simulink model "process_model_simulink"  (R2014b)
settings: Solver=ode45  StartTime=0.0  StopTime=500  RelTol=1e-3
values from neighbouring files (symbols this model uses):
  gs11_d = double(coeff_gs11(1))    [fase_minima.m]    (also in fase_nao_minima.m; model_minimum_phase.m; model_nonminimum_phase.m)
  gs11_ds = double(coeff_gs11(2))    [fase_minima.m]    (also in fase_nao_minima.m; model_minimum_phase.m; model_nonminimum_phase.m)
  gs11_n = gamma1*c1    [fase_minima.m]    (also in fase_nao_minima.m; model_minimum_phase.m; model_nonminimum_phase.m)
  gs12_d = double(coeff_gs12(1))    [fase_minima.m]    (also in fase_nao_minima.m; model_minimum_phase.m; model_nonminimum_phase.m)
  gs12_ds = double(coeff_gs12(2))    [fase_minima.m]    (also in fase_nao_minima.m; model_minimum_phase.m; model_nonminimum_phase.m)
  gs12_ds2 = double(coeff_gs12(3))    [fase_minima.m]    (also in fase_nao_minima.m; model_minimum_phase.m; model_nonminimum_phase.m)
  gs12_n = (1-gamma2)*c1    [fase_minima.m]    (also in fase_nao_minima.m; model_minimum_phase.m; model_nonminimum_phase.m)
  gs21_d = double(coeff_gs21(1))    [fase_minima.m]    (also in fase_nao_minima.m; model_minimum_phase.m; model_nonminimum_phase.m)
  gs21_ds = double(coeff_gs21(2))    [fase_minima.m]    (also in fase_nao_minima.m; model_minimum_phase.m; model_nonminimum_phase.m)
  gs21_ds2 = double(coeff_gs21(3))    [fase_minima.m]    (also in fase_nao_minima.m; model_minimum_phase.m; model_nonminimum_phase.m)
  gs21_n = (1-gamma1)*c2    [fase_minima.m]    (also in fase_nao_minima.m; model_minimum_phase.m; model_nonminimum_phase.m)
  gs22_d = double(coeff_gs22(1))    [fase_minima.m]    (also in fase_nao_minima.m; model_minimum_phase.m; model_nonminimum_phase.m)
  gs22_ds = double(coeff_gs22(2))    [fase_minima.m]    (also in fase_nao_minima.m; model_minimum_phase.m; model_nonminimum_phase.m)
  gs22_n = gamma2*c2    [fase_minima.m]    (also in fase_nao_minima.m; model_minimum_phase.m; model_nonminimum_phase.m)
settings Model: Creator=cfppwin  LastModifiedBy=cfppwin

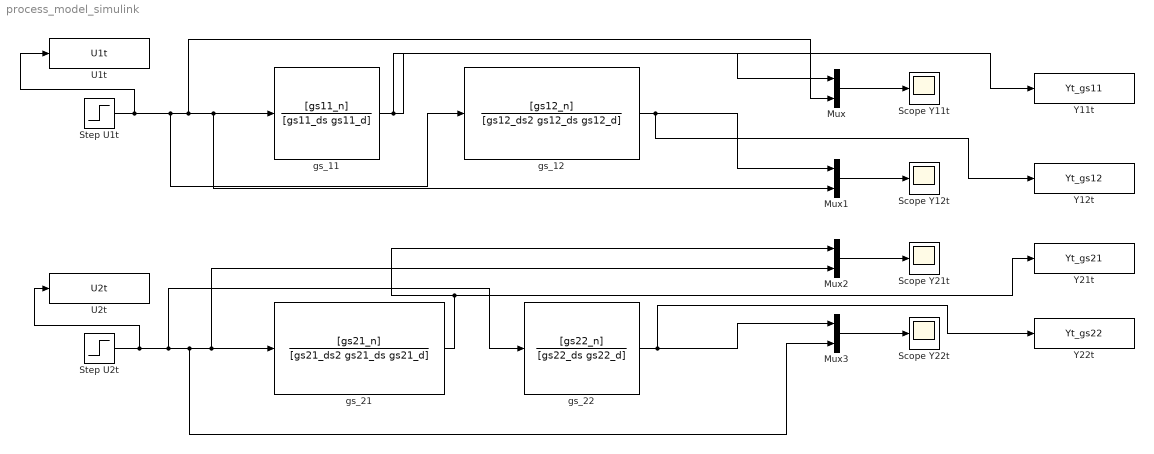
== system process_model_simulink ==
  Mux{,1..3} (4 alike) : Mux  Inputs=2
  Scope Y11t : Scope
      settings: ShowLegends=on  TimeRange=0.02452107279693294  YMin=0.01232600000000006  YMax=0.01264600000000007  ScrollMode=on
  Scope Y12t : Scope
      settings: ShowLegends=on  TimeRange=0.02452107279693294  YMin=0.01232600000000006  YMax=0.01264600000000007  ScrollMode=on
  Scope Y21t : Scope
      settings: ShowLegends=on  TimeRange=0.02452107279693294  YMin=0.01232600000000006  YMax=0.01264600000000007  SaveName=ScopeData2  ScrollMode=on
  Scope Y22t : Scope
      settings: ShowLegends=on  TimeRange=0.02452107279693294  YMin=0.01232600000000006  YMax=0.01264600000000007  SaveName=ScopeData3  ScrollMode=on
  Step U1t : Step  Time=50  SampleTime=0
  Step U2t : Step  Time=50  SampleTime=0
  U1t : ToWorkspace  VariableName=U1t  SampleTime=-1
      settings: Save2DSignal=2-D array (concatenate along first dimension)
  U2t : ToWorkspace  VariableName=U2t  SampleTime=-1
      settings: Save2DSignal=2-D array (concatenate along first dimension)
  Y11t : ToWorkspace  VariableName=Yt_gs11  SampleTime=-1
      settings: Save2DSignal=2-D array (concatenate along first dimension)
  Y12t : ToWorkspace  VariableName=Yt_gs12  SampleTime=-1
      settings: Save2DSignal=2-D array (concatenate along first dimension)
  Y21t : ToWorkspace  VariableName=Yt_gs21  SampleTime=-1
      settings: Save2DSignal=2-D array (concatenate along first dimension)
  Y22t : ToWorkspace  VariableName=Yt_gs22  SampleTime=-1
      settings: Save2DSignal=2-D array (concatenate along first dimension)
  gs_11 : TransferFcn  Numerator=[gs11_n]  Denominator=[gs11_ds gs11_d]
  gs_12 : TransferFcn  Numerator=[gs12_n]  Denominator=[gs12_ds2 gs12_ds gs12_d]
  "gs_21 " : TransferFcn  Numerator=[gs21_n]  Denominator=[gs21_ds2 gs21_ds gs21_d]
  gs_22 : TransferFcn  Numerator=[gs22_n]  Denominator=[gs22_ds gs22_d]
  wires:
  Step U1t/1 -> U1t/1, gs_12/1, Mux/2, Mux1/2, gs_11/1
  Step U2t/1 -> U2t/1, gs_22/1, Mux3/2, Mux2/2, "gs_21 "/1
  Mux/1 -> Scope Y11t/1
  Mux3/1 -> Scope Y22t/1
  Mux2/1 -> Scope Y21t/1
  Mux1/1 -> Scope Y12t/1
  gs_11/1 -> Y11t/1, Mux/1
  gs_12/1 -> Y12t/1, Mux1/1
  "gs_21 "/1 -> Mux2/1, Y21t/1
  gs_22/1 -> Y22t/1, Mux3/1
